simulink model "PSH_Coffee_SimulinkStateFlow_V2"  (R2018a)
settings: Solver=VariableStepAuto  StartTime=0.0  StopTime=200  FixedStep=0.01  RelTol=1e-3  EnableMultiTasking=on
settings Model: EnablePacing=on  PacingRate=0.500000  Creator=tunn  LastModifiedBy=tunn
settings SolverCC: AutoInsertRateTranBlk=on
settings OptimizationCC: LifeSpan=inf
settings DebuggingCC: SFUnexpectedBacktrackingDiag=warning  SFNoUnconditionalDefaultTransitionDiag=warning  SFExecutionAtInitializationDiag=none
settings CodeAppCC: StateflowObjectComments=on
settings GRTTargetCC: TargetLangStandard=C89/C90 (ANSI)
settings ConfigComp: CovMetricSettings=dw  CovHtmlReporting=on  CovSaveCumulativeToWorkspaceVar=on  CovSaveSingleToWorkspaceVar=on  CovShowResultsExplorer=off  CovExternalEMLEnable=off

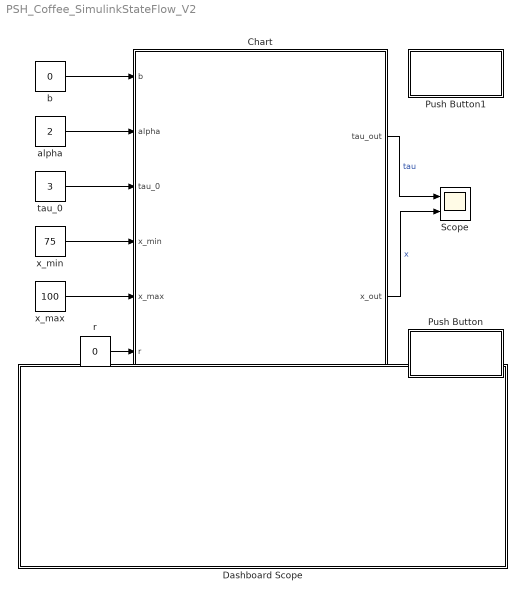
== system PSH_Coffee_SimulinkStateFlow_V2 ==
  Chart : Stateflow chart  TreatAsAtomicUnit=on
  Dashboard Scope : Subsystem  DialogController=hmiCreateDDGDialog  IsWebBlock=on  mask(MWDashboardBlock){webBlockId=0d24a4d6-6fd4-4889-9064-03b517be73d9, webBlockType=sdiscope, ShowInitialText=on, HMISrcModelName=PSH_Coffee_SimulinkStateFlow_V2}
      mask prompts: webBlockId "WebBlock Id"; webBlockType "WebBlock Type"; HMISrcModelName "Source Model"
      mask help: SimulinkHMI:dialogs:HMIScopeDialogDesc
      mask Help: helpview([docroot '/mapfiles/simulink.map'], 'hmi_scope')
      mask Display:
      | if strcmp(get_param(bdroot(gcb),'BlockDiagramType'), 'library')
      |     image([(matlabroot) '/toolbox/simulink/hmi/icons/DashboardScope.png']);
      | end
  Push Button : Subsystem  DialogController=hmiCreateDDGDialog  IsWebBlock=on  mask(MWDashboardBlock){webBlockId=8f9f16d7-94ec-48a8-890b-ffa68874c5a6, webBlockType=pushbutton, ShowInLibBrwoser=on, ShowInitialText=on, HMISrcModelName=PSH_Coffee_SimulinkStateFlow_V2}
      mask prompts: webBlockId "WebBlock Id"; webBlockType "WebBlock Type"; HMISrcModelName "Source Model"
      mask help: SimulinkHMI:dialogs:PushButtonDialogDesc
      mask Help: helpview([docroot '/mapfiles/simulink.map'], 'hmi_push_button')
      mask Display:
      | model = bdroot(gcb);
      | if strcmp(get_param(model,'BlockDiagramType'), 'library')
      |     image([(matlabroot) '/toolbox/simulink/hmi/icons/PushButton.png']);
      | end
  Push Button1 : Subsystem  DialogController=hmiCreateDDGDialog  IsWebBlock=on  mask(MWDashboardBlock){webBlockId=c0e5df00-5f3f-4258-b7d1-d7f3dc762040, webBlockType=pushbutton, ShowInLibBrwoser=on, ShowInitialText=on, HMISrcModelName=PSH_Coffee_SimulinkStateFlow_V2}
      mask prompts: webBlockId "WebBlock Id"; webBlockType "WebBlock Type"; HMISrcModelName "Source Model"
      mask help: SimulinkHMI:dialogs:PushButtonDialogDesc
      mask Help: helpview([docroot '/mapfiles/simulink.map'], 'hmi_push_button')
      mask Display:
      | model = bdroot(gcb);
      | if strcmp(get_param(model,'BlockDiagramType'), 'library')
      |     image([(matlabroot) '/toolbox/simulink/hmi/icons/PushButton.png']);
      | end
  Scope : Scope  NumInputPorts=2
  alpha : Constant  Value=2
  b : Constant  Value=0
  r : Constant  Value=0
  tau_0 : Constant  Value=3
  x_max : Constant  Value=100
  "x_min " : Constant  Value=75
  wires:
  b/1 -> Chart/1(b)
  alpha/1 -> Chart/2(alpha)
  tau_0/1 -> Chart/3(tau_0)
  Chart/1(tau_out) -> Scope/1  "tau"
  Chart/2(x_out) -> Scope/2  "x"
  "x_min "/1 -> Chart/4(x_min)
  x_max/1 -> Chart/5(x_max)
  r/1 -> Chart/6(r)

== system PSH_Coffee_SimulinkStateFlow_V2/Dashboard Scope ==

== system PSH_Coffee_SimulinkStateFlow_V2/Push Button ==

== system PSH_Coffee_SimulinkStateFlow_V2/Push Button1 ==

== stateflow chart PSH_Coffee_SimulinkStateFlow_V2/Chart ==
  settings: updateMethod=CONTINUOUS
  state On
    du:
    x_dot    = -alpha ;
    tau_dot =  1        ;
    x_out    = x         ;
    tau_out = tau      ;
  state Off
    du:
    x_dot    = 0    ;
    tau_dot = 0    ;
    x_out    = x     ;
    tau_out = tau ;
  (default) -> Off : {
      | x    = x_max ;
      | tau = 0         ;
      | }
  Off -> On [order 1] : [b && x > x_min]{tau = 0}
  On -> Off : [tau >= tau_0]
  Off -> Off [order 2] : [x <= x_min && r]{x = x_max}
  data: b input; alpha input; tau_0 input; x local; tau_out output; x_out output; tau local; x_min input; x_max input; r input
  data x settings: updateMethod=SF_CONTINUOUS_TIME_DATA
  data tau settings: updateMethod=SF_CONTINUOUS_TIME_DATA
